simulink model "FMDemodulationBlock"  (R2015a)
settings: Solver=ode45  StartTime=0.0  StopTime=1  MaxStep=0.0001  RelTol=1e-3
values from neighbouring files (symbols this model uses):
  fm = 20    [AMmain.m]    (also in FMmain.m = 10; PMmain.m = 10; main.m = 10)
libraries: dsparch4 x1, commsynccomp2 x1
settings Model: Creator=subed  LastModifiedBy=subed

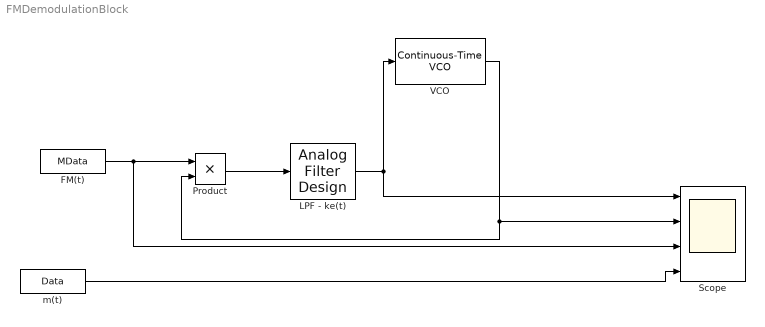
== system FMDemodulationBlock ==
  "FM(t) " : FromWorkspace  VariableName=MData  SampleTime=0
  "LPF - ke(t) " : dsparch4/Analog Filter Design  method=Butterworth  filttype=Lowpass  N=8  Wlo=2*pi*fm*2  Whi=80  Rp=1  Rs=40
  Product : Product
  Scope : Scope  NumInputPorts=4
      settings: ShowLegends=on  YMin=-5~-5~-5~-5  YMax=5~5~5~5
  "VCO " : commsynccomp2/Continuous-Time VCO  Ac=2  Fc=fc  Kc=10  Ph=0
  "m(t) " : FromWorkspace  VariableName=Data  SampleTime=0
  wires:
  Product/1 -> "LPF - ke(t) "/1
  "FM(t) "/1 -> Scope/3, Product/1
  "LPF - ke(t) "/1 -> Scope/1, "VCO "/1
  "VCO "/1 -> Scope/2, Product/2
  "m(t) "/1 -> Scope/4
